simulink model "Gen_net_5"  (R2018b)
settings: Solver=FixedStepAuto  StartTime=0.0  StopTime=100  FixedStep=0.1  RelTol=1e-3
undefined symbols (not defined in the file): g, Jx, Jy, Jz, m, phi_DoS_duration_1, phi_DoS_duration_2, phi_DoS_duration_3, phi_DoS_duration_4, phi_DoS_duration_5, phi_FDI_value_1, phi_FDI_value_2, phi_FDI_value_3, phi_FDI_value_4, phi_FDI_value_5, phi_Replay_delay_1, phi_Replay_delay_2, phi_Replay_delay_3, phi_Replay_delay_4, phi_Replay_delay_5, psi_DoS_duration_1, psi_DoS_duration_2, psi_DoS_duration_3, psi_DoS_duration_4, psi_DoS_duration_5, psi_FDI_value_1, psi_FDI_value_2, psi_FDI_value_3, psi_FDI_value_4, psi_FDI_value_5, psi_Replay_delay_1, psi_Replay_delay_2, psi_Replay_delay_3, psi_Replay_delay_4, psi_Replay_delay_5, T_DoS_duration_1, T_DoS_duration_2, T_DoS_duration_3, T_DoS_duration_4, T_DoS_duration_5, T_FDI_value_1, T_FDI_value_2, T_FDI_value_3, T_FDI_value_4, T_FDI_value_5, T_Replay_delay_1, T_Replay_delay_2, T_Replay_delay_3, T_Replay_delay_4, T_Replay_delay_5, tau_phi_DoS_duration_1, tau_phi_DoS_duration_2, tau_phi_DoS_duration_3, tau_phi_DoS_duration_4, tau_phi_DoS_duration_5, tau_phi_FDI_value_1, tau_phi_FDI_value_2, tau_phi_FDI_value_3, tau_phi_FDI_value_4, tau_phi_FDI_value_5 ... (+95)
libraries: simulink x30
(part 1 of 4)
settings Model: Creator=afsha  LastModifiedBy=afsha
settings DataIOCC: ReturnWorkspaceOutputs=on  ReturnWorkspaceOutputsName=logsout

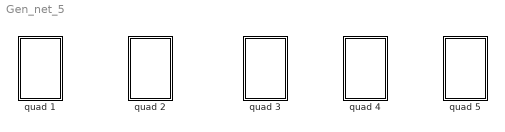
== system Gen_net_5 ==
  quad 1 : Subsystem
  quad 2 : Subsystem
  quad 3 : Subsystem
  quad 4 : Subsystem
  quad 5 : Subsystem

== system Gen_net_5/quad 1 ==
  actuator attack : Subsystem
  controller : Subsystem
  quadcopter : Subsystem
  references : Subsystem
  sensor attack : Subsystem
  wires:
  controller/4(tau_psi) -> actuator attack/4(tau_psi)  "tau_psi_1"
  quadcopter/4(phi) -> sensor attack/4(phi)  "phi"
  quadcopter/2(y) -> sensor attack/2(y)  "y"
  quadcopter/6(psi) -> sensor attack/6(psi)  "psi"
  references/2(y_ref) -> controller/2(y_ref)
  references/1(x_ref) -> controller/1(x_ref)
  controller/2(tau_phi) -> actuator attack/2(tau_phi)  "tau_phi_1"
  quadcopter/3(z) -> sensor attack/3(z)  "z"
  actuator attack/1(T_a) -> quadcopter/1(T)
  actuator attack/4(tau_psi_a) -> quadcopter/4(tau_psi)
  sensor attack/2(y_a) -> controller/5(y)  "y_a_1"
  sensor attack/4(phi_a) -> controller/7(phi)  "phi_a_1"
  quadcopter/1(x) -> sensor attack/1(x)  "x"
  actuator attack/3(tau_theta_a) -> quadcopter/3(tau_theta)
  sensor attack/5(theta_a) -> controller/8(theta)  "theta_a_1"
  sensor attack/6(psi_a) -> controller/9(psi)  "psi_a_1"
  controller/1(T) -> actuator attack/1(T)  "T_1"
  references/3(z_ref) -> controller/3(z_ref)
  controller/3(tau_theta) -> actuator attack/3(tau_theta)  "tau_theta_1"
  actuator attack/2(tau_phi_a) -> quadcopter/2(tau_ phi)
  sensor attack/1(x_a) -> controller/4(x)  "x_a_1"
  sensor attack/3(z_a) -> controller/6(z)  "z_a_1"
  quadcopter/5(theta) -> sensor attack/5(theta)  "theta"

== system Gen_net_5/quad 2 ==
  actuator attack : Subsystem
  controller : Subsystem
  quadcopter : Subsystem
  references : Subsystem
  sensor attack : Subsystem
  wires:
  controller/4(tau_psi) -> actuator attack/4(tau_psi)  "tau_psi_2"
  quadcopter/4(phi) -> sensor attack/4(phi)  "phi"
  quadcopter/2(y) -> sensor attack/2(y)  "y"
  quadcopter/6(psi) -> sensor attack/6(psi)  "psi"
  references/2(y_ref) -> controller/2(y_ref)
  references/1(x_ref) -> controller/1(x_ref)
  controller/2(tau_phi) -> actuator attack/2(tau_phi)  "tau_phi_2"
  quadcopter/3(z) -> sensor attack/3(z)  "z"
  actuator attack/1(T_a) -> quadcopter/1(T)
  actuator attack/4(tau_psi_a) -> quadcopter/4(tau_psi)
  sensor attack/2(y_a) -> controller/5(y)  "y_a_2"
  sensor attack/4(phi_a) -> controller/7(phi)  "phi_a_2"
  quadcopter/1(x) -> sensor attack/1(x)  "x"
  actuator attack/3(tau_theta_a) -> quadcopter/3(tau_theta)
  sensor attack/5(theta_a) -> controller/8(theta)  "theta_a_2"
  sensor attack/6(psi_a) -> controller/9(psi)  "psi_a_2"
  controller/1(T) -> actuator attack/1(T)  "T_2"
  references/3(z_ref) -> controller/3(z_ref)
  controller/3(tau_theta) -> actuator attack/3(tau_theta)  "tau_theta_2"
  actuator attack/2(tau_phi_a) -> quadcopter/2(tau_ phi)
  sensor attack/1(x_a) -> controller/4(x)  "x_a_2"
  sensor attack/3(z_a) -> controller/6(z)  "z_a_2"
  quadcopter/5(theta) -> sensor attack/5(theta)  "theta"

== system Gen_net_5/quad 3 ==
  actuator attack : Subsystem
  controller : Subsystem
  quadcopter : Subsystem
  references : Subsystem
  sensor attack : Subsystem
  wires:
  controller/4(tau_psi) -> actuator attack/4(tau_psi)  "tau_psi_3"
  quadcopter/4(phi) -> sensor attack/4(phi)  "phi"
  quadcopter/2(y) -> sensor attack/2(y)  "y"
  quadcopter/6(psi) -> sensor attack/6(psi)  "psi"
  references/2(y_ref) -> controller/2(y_ref)
  references/1(x_ref) -> controller/1(x_ref)
  controller/2(tau_phi) -> actuator attack/2(tau_phi)  "tau_phi_3"
  quadcopter/3(z) -> sensor attack/3(z)  "z"
  actuator attack/1(T_a) -> quadcopter/1(T)
  actuator attack/4(tau_psi_a) -> quadcopter/4(tau_psi)
  sensor attack/2(y_a) -> controller/5(y)  "y_a_3"
  sensor attack/4(phi_a) -> controller/7(phi)  "phi_a_3"
  quadcopter/1(x) -> sensor attack/1(x)  "x"
  actuator attack/3(tau_theta_a) -> quadcopter/3(tau_theta)
  sensor attack/5(theta_a) -> controller/8(theta)  "theta_a_3"
  sensor attack/6(psi_a) -> controller/9(psi)  "psi_a_3"
  controller/1(T) -> actuator attack/1(T)  "T_3"
  references/3(z_ref) -> controller/3(z_ref)
  controller/3(tau_theta) -> actuator attack/3(tau_theta)  "tau_theta_3"
  actuator attack/2(tau_phi_a) -> quadcopter/2(tau_ phi)
  sensor attack/1(x_a) -> controller/4(x)  "x_a_3"
  sensor attack/3(z_a) -> controller/6(z)  "z_a_3"
  quadcopter/5(theta) -> sensor attack/5(theta)  "theta"

== system Gen_net_5/quad 4 ==
  actuator attack : Subsystem
  controller : Subsystem
  quadcopter : Subsystem
  references : Subsystem
  sensor attack : Subsystem
  wires:
  controller/4(tau_psi) -> actuator attack/4(tau_psi)  "tau_psi_4"
  quadcopter/4(phi) -> sensor attack/4(phi)  "phi"
  quadcopter/2(y) -> sensor attack/2(y)  "y"
  quadcopter/6(psi) -> sensor attack/6(psi)  "psi"
  references/2(y_ref) -> controller/2(y_ref)
  references/1(x_ref) -> controller/1(x_ref)
  controller/2(tau_phi) -> actuator attack/2(tau_phi)  "tau_phi_4"
  quadcopter/3(z) -> sensor attack/3(z)  "z"
  actuator attack/1(T_a) -> quadcopter/1(T)
  actuator attack/4(tau_psi_a) -> quadcopter/4(tau_psi)
  sensor attack/2(y_a) -> controller/5(y)  "y_a_4"
  sensor attack/4(phi_a) -> controller/7(phi)  "phi_a_4"
  quadcopter/1(x) -> sensor attack/1(x)  "x"
  actuator attack/3(tau_theta_a) -> quadcopter/3(tau_theta)
  sensor attack/5(theta_a) -> controller/8(theta)  "theta_a_4"
  sensor attack/6(psi_a) -> controller/9(psi)  "psi_a_4"
  controller/1(T) -> actuator attack/1(T)  "T_4"
  references/3(z_ref) -> controller/3(z_ref)
  controller/3(tau_theta) -> actuator attack/3(tau_theta)  "tau_theta_4"
  actuator attack/2(tau_phi_a) -> quadcopter/2(tau_ phi)
  sensor attack/1(x_a) -> controller/4(x)  "x_a_4"
  sensor attack/3(z_a) -> controller/6(z)  "z_a_4"
  quadcopter/5(theta) -> sensor attack/5(theta)  "theta"

== system Gen_net_5/quad 5 ==
  actuator attack : Subsystem
  controller : Subsystem
  quadcopter : Subsystem
  references : Subsystem
  sensor attack : Subsystem
  wires:
  controller/4(tau_psi) -> actuator attack/4(tau_psi)  "tau_psi_5"
  quadcopter/4(phi) -> sensor attack/4(phi)  "phi"
  quadcopter/2(y) -> sensor attack/2(y)  "y"
  quadcopter/6(psi) -> sensor attack/6(psi)  "psi"
  references/2(y_ref) -> controller/2(y_ref)
  references/1(x_ref) -> controller/1(x_ref)
  controller/2(tau_phi) -> actuator attack/2(tau_phi)  "tau_phi_5"
  quadcopter/3(z) -> sensor attack/3(z)  "z"
  actuator attack/1(T_a) -> quadcopter/1(T)
  actuator attack/4(tau_psi_a) -> quadcopter/4(tau_psi)
  sensor attack/2(y_a) -> controller/5(y)  "y_a_5"
  sensor attack/4(phi_a) -> controller/7(phi)  "phi_a_5"
  quadcopter/1(x) -> sensor attack/1(x)  "x"
  actuator attack/3(tau_theta_a) -> quadcopter/3(tau_theta)
  sensor attack/5(theta_a) -> controller/8(theta)  "theta_a_5"
  sensor attack/6(psi_a) -> controller/9(psi)  "psi_a_5"
  controller/1(T) -> actuator attack/1(T)  "T_5"
  references/3(z_ref) -> controller/3(z_ref)
  controller/3(tau_theta) -> actuator attack/3(tau_theta)  "tau_theta_5"
  actuator attack/2(tau_phi_a) -> quadcopter/2(tau_ phi)
  sensor attack/1(x_a) -> controller/4(x)  "x_a_5"
  sensor attack/3(z_a) -> controller/6(z)  "z_a_5"
  quadcopter/5(theta) -> sensor attack/5(theta)  "theta"

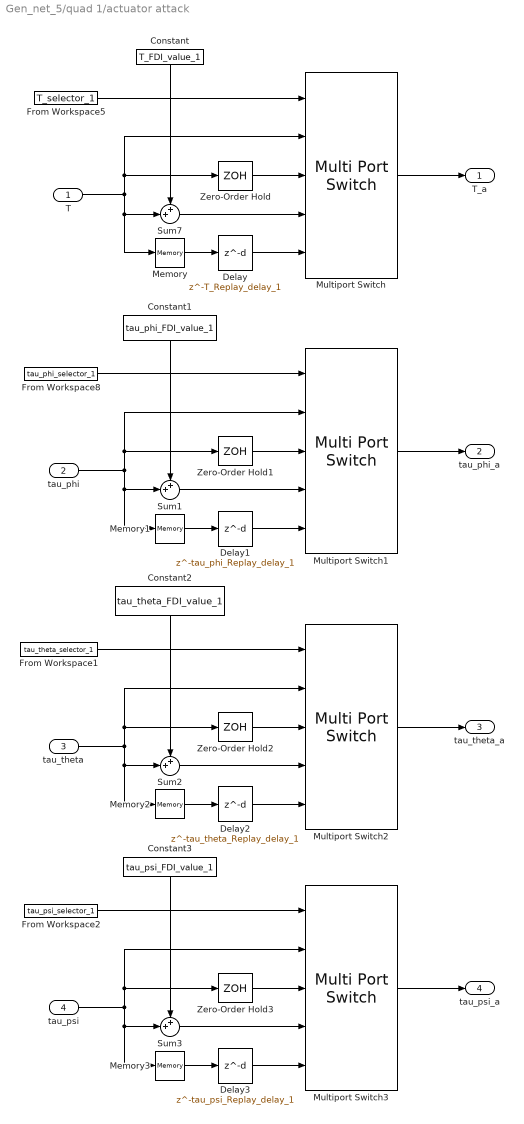
== system Gen_net_5/quad 1/actuator attack ==
  T : Inport
  tau_phi : Inport  Port=2
  tau_theta : Inport  Port=3
  tau_psi : Inport  Port=4
  Constant : Constant  Value=T_FDI_value_1
  Constant1 : Constant  Value=tau_phi_FDI_value_1
  Constant2 : Constant  Value=tau_theta_FDI_value_1
  Constant3 : Constant  Value=tau_psi_FDI_value_1
  Delay : Delay  DelayLength=T_Replay_delay_1  DelayLengthUpperLimit=40
  Delay1 : Delay  DelayLength=tau_phi_Replay_delay_1  DelayLengthUpperLimit=40
  Delay2 : Delay  DelayLength=tau_theta_Replay_delay_1  DelayLengthUpperLimit=40
  Delay3 : Delay  DelayLength=tau_psi_Replay_delay_1  DelayLengthUpperLimit=40
  From Workspace1 : FromWorkspace  VariableName=tau_theta_selector_1  SampleTime=0
  From Workspace2 : FromWorkspace  VariableName=tau_psi_selector_1  SampleTime=0
  From Workspace5 : FromWorkspace  VariableName=T_selector_1  SampleTime=0
  From Workspace8 : FromWorkspace  VariableName=tau_phi_selector_1  SampleTime=0
  Memory{,1..3} (4 alike) : Memory
  Multiport Switch{,1..3} (4 alike) : MultiPortSwitch  Inputs=4
  Sum{1..3,7} (4 alike) : Sum  Inputs=++|
  Zero-Order Hold : ZeroOrderHold  SampleTime=T_DoS_duration_1
  Zero-Order Hold1 : ZeroOrderHold  SampleTime=tau_phi_DoS_duration_1
  Zero-Order Hold2 : ZeroOrderHold  SampleTime=tau_theta_DoS_duration_1
  Zero-Order Hold3 : ZeroOrderHold  SampleTime=tau_psi_DoS_duration_1
  T_a : Outport
  tau_phi_a : Outport  Port=2
  tau_theta_a : Outport  Port=3
  tau_psi_a : Outport  Port=4
  wires:
  T/1 -> Sum7/2, Memory/1, Multiport Switch/2, Zero-Order Hold/1
  Zero-Order Hold/1 -> Multiport Switch/3
  Sum7/1 -> Multiport Switch/4
  From Workspace5/1 -> Multiport Switch/1
  Multiport Switch/1 -> T_a/1
  Memory/1 -> Delay/1
  Constant/1 -> Sum7/1
  Delay/1 -> Multiport Switch/5
  Memory1/1 -> Delay1/1
  Delay1/1 -> Multiport Switch1/5
  Zero-Order Hold1/1 -> Multiport Switch1/3
  Constant1/1 -> Sum1/1
  Sum1/1 -> Multiport Switch1/4
  Multiport Switch1/1 -> tau_phi_a/1
  tau_phi/1 -> Sum1/2, Memory1/1, Multiport Switch1/2, Zero-Order Hold1/1
  From Workspace8/1 -> Multiport Switch1/1
  Memory2/1 -> Delay2/1
  Delay2/1 -> Multiport Switch2/5
  Zero-Order Hold2/1 -> Multiport Switch2/3
  Constant2/1 -> Sum2/1
  Sum2/1 -> Multiport Switch2/4
  Multiport Switch2/1 -> tau_theta_a/1
  tau_theta/1 -> Sum2/2, Memory2/1, Multiport Switch2/2, Zero-Order Hold2/1
  From Workspace1/1 -> Multiport Switch2/1
  Memory3/1 -> Delay3/1
  Delay3/1 -> Multiport Switch3/5
  Zero-Order Hold3/1 -> Multiport Switch3/3
  Constant3/1 -> Sum3/1
  Sum3/1 -> Multiport Switch3/4
  Multiport Switch3/1 -> tau_psi_a/1
  tau_psi/1 -> Sum3/2, Memory3/1, Multiport Switch3/2, Zero-Order Hold3/1
  From Workspace2/1 -> Multiport Switch3/1

== system Gen_net_5/quad 1/controller ==
  x_ref : Inport
  y_ref : Inport  Port=2
  z_ref : Inport  Port=3
  x : Inport  Port=4
  y : Inport  Port=5
  z : Inport  Port=6
  phi : Inport  Port=7
  theta : Inport  Port=8
  psi : Inport  Port=9
  altitude controller : Subsystem
  attitude controller : Subsystem
  position controller : Subsystem
  yaw controller : Subsystem
  T : Outport
  tau_phi : Outport  Port=2
  tau_theta : Outport  Port=3
  tau_psi : Outport  Port=4
  wires:
  yaw controller/1(tau_psi) -> tau_psi/1
  phi/1 -> attitude controller/1(phi)
  y_ref/1 -> position controller/3(y_ref)
  x/1 -> position controller/2(x)
  position controller/2(theta_ref) -> attitude controller/4(theta_ref)
  position controller/1(phi_ref) -> attitude controller/3(phi_ref)
  x_ref/1 -> position controller/1(x_ref)
  attitude controller/1(tau_phi) -> tau_phi/1
  y/1 -> position controller/4(y)
  psi/1 -> yaw controller/1(yaw)
  attitude controller/2(tau_theta) -> tau_theta/1
  theta/1 -> attitude controller/2(theta)
  z_ref/1 -> altitude controller/1(z_ref)
  altitude controller/1(T) -> T/1
  z/1 -> altitude controller/2(z)

== system Gen_net_5/quad 1/quadcopter ==
  T : Inport
  tau_ phi : Inport  Port=2
  tau_theta : Inport  Port=3
  tau_psi : Inport  Port=4
  Demux : Demux  Outputs=12
  Demux1 : Demux  Outputs=12
  Gain : Gain  Gain=1/m
  Integrator12 : Integrator
  Mux : Mux  Inputs=12
  S(10-12) : Subsystem
  S(4-6) : Subsystem
  S(7-9) : Subsystem
  Scope1 : Scope  NumInputPorts=3
  Scope2 : Scope  NumInputPorts=3
  Terminator : Terminator
  Terminator1 : Terminator
  Terminator2 : Terminator
  angle : Scope  NumInputPorts=3
  position : Scope  NumInputPorts=3
  x : Outport
  y : Outport  Port=2
  z : Outport  Port=3
  phi : Outport  Port=4
  theta : Outport  Port=5
  psi : Outport  Port=6
  wires:
  Mux/1 -> Integrator12/1
  Integrator12/1 -> Demux/1, Demux1/1
  Demux/2 -> position/2, y/1  "y"
  Demux/3 -> z/1, position/3  "z"
  Demux/1 -> x/1, position/1  "x"
  Demux/5 -> Scope1/2  "Vy"
  Demux/4 -> Scope1/1  "Vx"
  Demux/6 -> Scope1/3  "Vz"
  Demux/8 -> angle/2, theta/1  "theta"
  Demux/7 -> angle/1, phi/1  "phi"
  Demux/9 -> angle/3, psi/1  "psi"
  Demux/12 -> Scope2/3  "r"
  Demux/10 -> Scope2/1  "p"
  Demux/11 -> Scope2/2  "q"
  Demux1/4 -> Mux/1  "Vx"
  Demux1/5 -> Mux/2  "Vy"
  Demux1/6 -> Mux/3  "Vz"
  Demux1/8 -> S(4-6)/3(theta), S(7-9)/2(theta)  "theta"
  Demux1/7 -> S(4-6)/2(phi), S(7-9)/1(phi)  "phi"
  Demux1/10 -> S(10-12)/2(P), S(7-9)/4(P)  "P"
  Demux1/11 -> S(7-9)/3(q), S(10-12)/1(q)  "q"
  Demux1/12 -> S(7-9)/5(r), S(10-12)/3(r)
  Gain/1 -> S(4-6)/1(In1)
  Demux1/9 -> S(4-6)/4(psi)  "psi"
  S(4-6)/1(Out1) -> Mux/4
  S(4-6)/2(Out2) -> Mux/5
  S(4-6)/3(Out3) -> Mux/6
  S(7-9)/1(Out1) -> Mux/7
  S(7-9)/2(Out2) -> Mux/8
  S(7-9)/3(Out3) -> Mux/9
  tau_ phi/1 -> S(10-12)/4(In4)
  tau_theta/1 -> S(10-12)/5(In5)
  tau_psi/1 -> S(10-12)/6(In6)
  S(10-12)/1(Out1) -> Mux/10
  S(10-12)/2(Out2) -> Mux/11
  S(10-12)/3(Out3) -> Mux/12
  Demux1/1 -> Terminator/1  "x"
  Demux1/2 -> Terminator1/1  "y"
  Demux1/3 -> Terminator2/1  "z"
  T/1 -> Gain/1  "z_ref"

== system Gen_net_5/quad 1/references ==
  From Workspace : FromWorkspace  VariableName=z_ref_1  SampleTime=0
  From Workspace1 : FromWorkspace  VariableName=x_ref_1  SampleTime=0
  From Workspace2 : FromWorkspace  VariableName=y_ref_1  SampleTime=0
  reference : Scope  NumInputPorts=3
  x_ref : Outport
  y_ref : Outport  Port=2
  z_ref : Outport  Port=3
  wires:
  From Workspace1/1 -> reference/1, x_ref/1  "x_ref"
  From Workspace/1 -> reference/3, z_ref/1  "z_ref"
  From Workspace2/1 -> reference/2, y_ref/1  "y_ref"

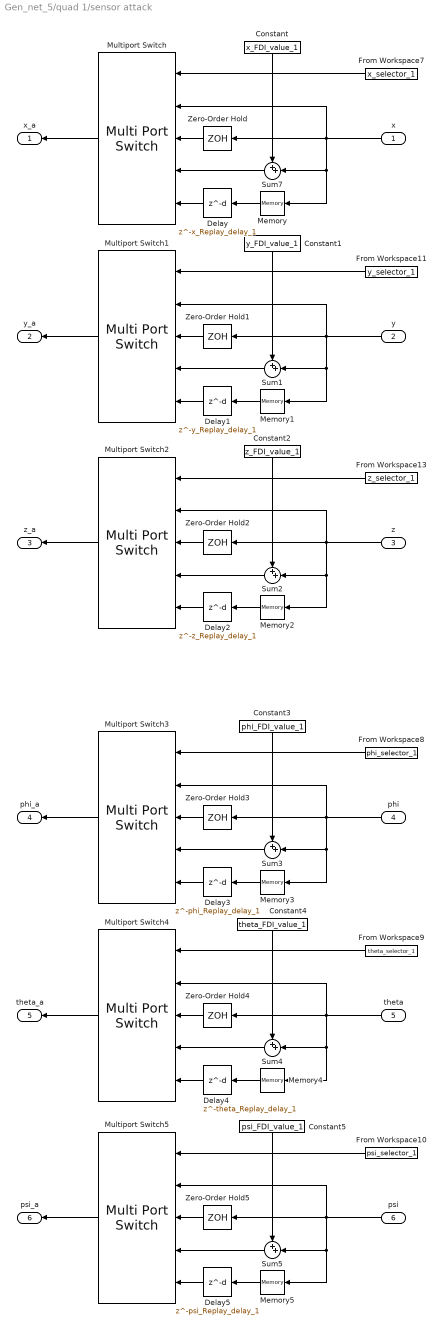
== system Gen_net_5/quad 1/sensor attack ==
  x : Inport
  y : Inport  Port=2
  z : Inport  Port=3
  phi : Inport  Port=4
  theta : Inport  Port=5
  psi : Inport  Port=6
  Constant : Constant  Value=x_FDI_value_1
  Constant1 : Constant  Value=y_FDI_value_1
  Constant2 : Constant  Value=z_FDI_value_1
  Constant3 : Constant  Value=phi_FDI_value_1
  Constant4 : Constant  Value=theta_FDI_value_1
  Constant5 : Constant  Value=psi_FDI_value_1
  Delay : Delay  DelayLength=x_Replay_delay_1  DelayLengthUpperLimit=40
  Delay1 : Delay  DelayLength=y_Replay_delay_1  DelayLengthUpperLimit=40
  Delay2 : Delay  DelayLength=z_Replay_delay_1  DelayLengthUpperLimit=40
  Delay3 : Delay  DelayLength=phi_Replay_delay_1  DelayLengthUpperLimit=40
  Delay4 : Delay  DelayLength=theta_Replay_delay_1  DelayLengthUpperLimit=40
  Delay5 : Delay  DelayLength=psi_Replay_delay_1  DelayLengthUpperLimit=40
  From Workspace10 : FromWorkspace  VariableName=psi_selector_1  SampleTime=0
  From Workspace11 : FromWorkspace  VariableName=y_selector_1  SampleTime=0
  From Workspace13 : FromWorkspace  VariableName=z_selector_1  SampleTime=0
  From Workspace7 : FromWorkspace  VariableName=x_selector_1  SampleTime=0
  From Workspace8 : FromWorkspace  VariableName=phi_selector_1  SampleTime=0
  From Workspace9 : FromWorkspace  VariableName=theta_selector_1  SampleTime=0
  Memory{,1..5} (6 alike) : Memory
  Multiport Switch{,1..5} (6 alike) : MultiPortSwitch  Inputs=4
  Sum{1..5,7} (6 alike) : Sum  Inputs=++|
  Zero-Order Hold : ZeroOrderHold  SampleTime=x_DoS_duration_1
  Zero-Order Hold1 : ZeroOrderHold  SampleTime=y_DoS_duration_1
  Zero-Order Hold2 : ZeroOrderHold  SampleTime=z_DoS_duration_1
  Zero-Order Hold3 : ZeroOrderHold  SampleTime=phi_DoS_duration_1
  Zero-Order Hold4 : ZeroOrderHold  SampleTime=theta_DoS_duration_1
  Zero-Order Hold5 : ZeroOrderHold  SampleTime=psi_DoS_duration_1
  x_a : Outport
  y_a : Outport  Port=2
  z_a : Outport  Port=3
  phi_a : Outport  Port=4
  theta_a : Outport  Port=5
  psi_a : Outport  Port=6
  wires:
  Memory/1 -> Delay/1
  Delay/1 -> Multiport Switch/5
  Zero-Order Hold/1 -> Multiport Switch/3
  Constant/1 -> Sum7/1
  Sum7/1 -> Multiport Switch/4
  Multiport Switch/1 -> x_a/1
  x/1 -> Multiport Switch/2, Zero-Order Hold/1, Sum7/2, Memory/1
  From Workspace7/1 -> Multiport Switch/1
  From Workspace11/1 -> Multiport Switch1/1
  Sum1/1 -> Multiport Switch1/4
  Delay1/1 -> Multiport Switch1/5
  Constant1/1 -> Sum1/1
  Memory1/1 -> Delay1/1
  y/1 -> Multiport Switch1/2, Zero-Order Hold1/1, Sum1/2, Memory1/1
  Multiport Switch1/1 -> y_a/1
  Zero-Order Hold1/1 -> Multiport Switch1/3
  From Workspace13/1 -> Multiport Switch2/1
  Sum2/1 -> Multiport Switch2/4
  Delay2/1 -> Multiport Switch2/5
  Constant2/1 -> Sum2/1
  Memory2/1 -> Delay2/1
  z/1 -> Multiport Switch2/2, Zero-Order Hold2/1, Sum2/2, Memory2/1
  Multiport Switch2/1 -> z_a/1
  Zero-Order Hold2/1 -> Multiport Switch2/3
  From Workspace8/1 -> Multiport Switch3/1
  Sum3/1 -> Multiport Switch3/4
  Delay3/1 -> Multiport Switch3/5
  Constant3/1 -> Sum3/1
  Memory3/1 -> Delay3/1
  phi/1 -> Multiport Switch3/2, Zero-Order Hold3/1, Sum3/2, Memory3/1
  Multiport Switch3/1 -> phi_a/1
  Zero-Order Hold3/1 -> Multiport Switch3/3
  From Workspace9/1 -> Multiport Switch4/1
  Sum4/1 -> Multiport Switch4/4
  Delay4/1 -> Multiport Switch4/5
  Constant4/1 -> Sum4/1
  Memory4/1 -> Delay4/1
  theta/1 -> Multiport Switch4/2, Zero-Order Hold4/1, Sum4/2, Memory4/1
  Multiport Switch4/1 -> theta_a/1
  Zero-Order Hold4/1 -> Multiport Switch4/3
  From Workspace10/1 -> Multiport Switch5/1
  Sum5/1 -> Multiport Switch5/4
  Delay5/1 -> Multiport Switch5/5
  Constant5/1 -> Sum5/1
  Memory5/1 -> Delay5/1
  psi/1 -> Multiport Switch5/2, Zero-Order Hold5/1, Sum5/2, Memory5/1
  Multiport Switch5/1 -> psi_a/1
  Zero-Order Hold5/1 -> Multiport Switch5/3

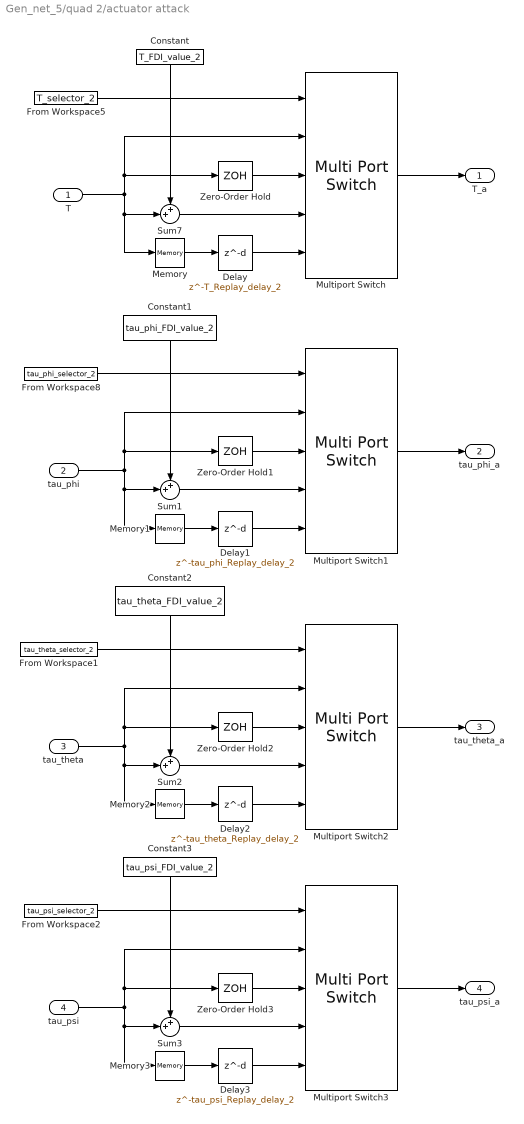
== system Gen_net_5/quad 2/actuator attack ==
  T : Inport
  tau_phi : Inport  Port=2
  tau_theta : Inport  Port=3
  tau_psi : Inport  Port=4
  Constant : Constant  Value=T_FDI_value_2
  Constant1 : Constant  Value=tau_phi_FDI_value_2
  Constant2 : Constant  Value=tau_theta_FDI_value_2
  Constant3 : Constant  Value=tau_psi_FDI_value_2
  Delay : Delay  DelayLength=T_Replay_delay_2  DelayLengthUpperLimit=40
  Delay1 : Delay  DelayLength=tau_phi_Replay_delay_2  DelayLengthUpperLimit=40
  Delay2 : Delay  DelayLength=tau_theta_Replay_delay_2  DelayLengthUpperLimit=40
  Delay3 : Delay  DelayLength=tau_psi_Replay_delay_2  DelayLengthUpperLimit=40
  From Workspace1 : FromWorkspace  VariableName=tau_theta_selector_2  SampleTime=0
  From Workspace2 : FromWorkspace  VariableName=tau_psi_selector_2  SampleTime=0
  From Workspace5 : FromWorkspace  VariableName=T_selector_2  SampleTime=0
  From Workspace8 : FromWorkspace  VariableName=tau_phi_selector_2  SampleTime=0
  Memory{,1..3} (4 alike) : Memory
  Multiport Switch{,1..3} (4 alike) : MultiPortSwitch  Inputs=4
  Sum{1..3,7} (4 alike) : Sum  Inputs=++|
  Zero-Order Hold : ZeroOrderHold  SampleTime=T_DoS_duration_2
  Zero-Order Hold1 : ZeroOrderHold  SampleTime=tau_phi_DoS_duration_2
  Zero-Order Hold2 : ZeroOrderHold  SampleTime=tau_theta_DoS_duration_2
  Zero-Order Hold3 : ZeroOrderHold  SampleTime=tau_psi_DoS_duration_2
  T_a : Outport
  tau_phi_a : Outport  Port=2
  tau_theta_a : Outport  Port=3
  tau_psi_a : Outport  Port=4
  wires:
  T/1 -> Sum7/2, Memory/1, Multiport Switch/2, Zero-Order Hold/1
  Zero-Order Hold/1 -> Multiport Switch/3
  Sum7/1 -> Multiport Switch/4
  From Workspace5/1 -> Multiport Switch/1
  Multiport Switch/1 -> T_a/1
  Memory/1 -> Delay/1
  Constant/1 -> Sum7/1
  Delay/1 -> Multiport Switch/5
  Memory1/1 -> Delay1/1
  Delay1/1 -> Multiport Switch1/5
  Zero-Order Hold1/1 -> Multiport Switch1/3
  Constant1/1 -> Sum1/1
  Sum1/1 -> Multiport Switch1/4
  Multiport Switch1/1 -> tau_phi_a/1
  tau_phi/1 -> Sum1/2, Memory1/1, Multiport Switch1/2, Zero-Order Hold1/1
  From Workspace8/1 -> Multiport Switch1/1
  Memory2/1 -> Delay2/1
  Delay2/1 -> Multiport Switch2/5
  Zero-Order Hold2/1 -> Multiport Switch2/3
  Constant2/1 -> Sum2/1
  Sum2/1 -> Multiport Switch2/4
  Multiport Switch2/1 -> tau_theta_a/1
  tau_theta/1 -> Sum2/2, Memory2/1, Multiport Switch2/2, Zero-Order Hold2/1
  From Workspace1/1 -> Multiport Switch2/1
  Memory3/1 -> Delay3/1
  Delay3/1 -> Multiport Switch3/5
  Zero-Order Hold3/1 -> Multiport Switch3/3
  Constant3/1 -> Sum3/1
  Sum3/1 -> Multiport Switch3/4
  Multiport Switch3/1 -> tau_psi_a/1
  tau_psi/1 -> Sum3/2, Memory3/1, Multiport Switch3/2, Zero-Order Hold3/1
  From Workspace2/1 -> Multiport Switch3/1

== system Gen_net_5/quad 2/controller ==
  x_ref : Inport
  y_ref : Inport  Port=2
  z_ref : Inport  Port=3
  x : Inport  Port=4
  y : Inport  Port=5
  z : Inport  Port=6
  phi : Inport  Port=7
  theta : Inport  Port=8
  psi : Inport  Port=9
  altitude controller : Subsystem
  attitude controller : Subsystem
  position controller : Subsystem
  yaw controller : Subsystem
  T : Outport
  tau_phi : Outport  Port=2
  tau_theta : Outport  Port=3
  tau_psi : Outport  Port=4
  wires:
  yaw controller/1(tau_psi) -> tau_psi/1
  phi/1 -> attitude controller/1(phi)
  y_ref/1 -> position controller/3(y_ref)
  x/1 -> position controller/2(x)
  position controller/2(theta_ref) -> attitude controller/4(theta_ref)
  position controller/1(phi_ref) -> attitude controller/3(phi_ref)
  x_ref/1 -> position controller/1(x_ref)
  attitude controller/1(tau_phi) -> tau_phi/1
  y/1 -> position controller/4(y)
  psi/1 -> yaw controller/1(yaw)
  attitude controller/2(tau_theta) -> tau_theta/1
  theta/1 -> attitude controller/2(theta)
  z_ref/1 -> altitude controller/1(z_ref)
  altitude controller/1(T) -> T/1
  z/1 -> altitude controller/2(z)

== system Gen_net_5/quad 2/quadcopter ==
  T : Inport
  tau_ phi : Inport  Port=2
  tau_theta : Inport  Port=3
  tau_psi : Inport  Port=4
  Demux : Demux  Outputs=12
  Demux1 : Demux  Outputs=12
  Gain : Gain  Gain=1/m
  Integrator12 : Integrator
  Mux : Mux  Inputs=12
  S(10-12) : Subsystem
  S(4-6) : Subsystem
  S(7-9) : Subsystem
  Scope1 : Scope  NumInputPorts=3
  Scope2 : Scope  NumInputPorts=3
  Terminator : Terminator
  Terminator1 : Terminator
  Terminator2 : Terminator
  angle : Scope  NumInputPorts=3
  position : Scope  NumInputPorts=3
  x : Outport
  y : Outport  Port=2
  z : Outport  Port=3
  phi : Outport  Port=4
  theta : Outport  Port=5
  psi : Outport  Port=6
  wires:
  Mux/1 -> Integrator12/1
  Integrator12/1 -> Demux/1, Demux1/1
  Demux/2 -> position/2, y/1  "y"
  Demux/3 -> z/1, position/3  "z"
  Demux/1 -> x/1, position/1  "x"
  Demux/5 -> Scope1/2  "Vy"
  Demux/4 -> Scope1/1  "Vx"
  Demux/6 -> Scope1/3  "Vz"
  Demux/8 -> angle/2, theta/1  "theta"
  Demux/7 -> angle/1, phi/1  "phi"
  Demux/9 -> angle/3, psi/1  "psi"
  Demux/12 -> Scope2/3  "r"
  Demux/10 -> Scope2/1  "p"
  Demux/11 -> Scope2/2  "q"
  Demux1/4 -> Mux/1  "Vx"
  Demux1/5 -> Mux/2  "Vy"
  Demux1/6 -> Mux/3  "Vz"
  Demux1/8 -> S(4-6)/3(theta), S(7-9)/2(theta)  "theta"
  Demux1/7 -> S(4-6)/2(phi), S(7-9)/1(phi)  "phi"
  Demux1/10 -> S(10-12)/2(P), S(7-9)/4(P)  "P"
  Demux1/11 -> S(7-9)/3(q), S(10-12)/1(q)  "q"
  Demux1/12 -> S(7-9)/5(r), S(10-12)/3(r)
  Gain/1 -> S(4-6)/1(In1)
  Demux1/9 -> S(4-6)/4(psi)  "psi"
  S(4-6)/1(Out1) -> Mux/4
  S(4-6)/2(Out2) -> Mux/5
  S(4-6)/3(Out3) -> Mux/6
  S(7-9)/1(Out1) -> Mux/7
  S(7-9)/2(Out2) -> Mux/8
  S(7-9)/3(Out3) -> Mux/9
  tau_ phi/1 -> S(10-12)/4(In4)
  tau_theta/1 -> S(10-12)/5(In5)
  tau_psi/1 -> S(10-12)/6(In6)
  S(10-12)/1(Out1) -> Mux/10
  S(10-12)/2(Out2) -> Mux/11
  S(10-12)/3(Out3) -> Mux/12
  Demux1/1 -> Terminator/1  "x"
  Demux1/2 -> Terminator1/1  "y"
  Demux1/3 -> Terminator2/1  "z"
  T/1 -> Gain/1  "z_ref"

== system Gen_net_5/quad 2/references ==
  From Workspace : FromWorkspace  VariableName=z_ref_2  SampleTime=0
  From Workspace1 : FromWorkspace  VariableName=x_ref_2  SampleTime=0
  From Workspace2 : FromWorkspace  VariableName=y_ref_2  SampleTime=0
  reference : Scope  NumInputPorts=3
  x_ref : Outport
  y_ref : Outport  Port=2
  z_ref : Outport  Port=3
  wires:
  From Workspace1/1 -> reference/1, x_ref/1  "x_ref"
  From Workspace/1 -> reference/3, z_ref/1  "z_ref"
  From Workspace2/1 -> reference/2, y_ref/1  "y_ref"

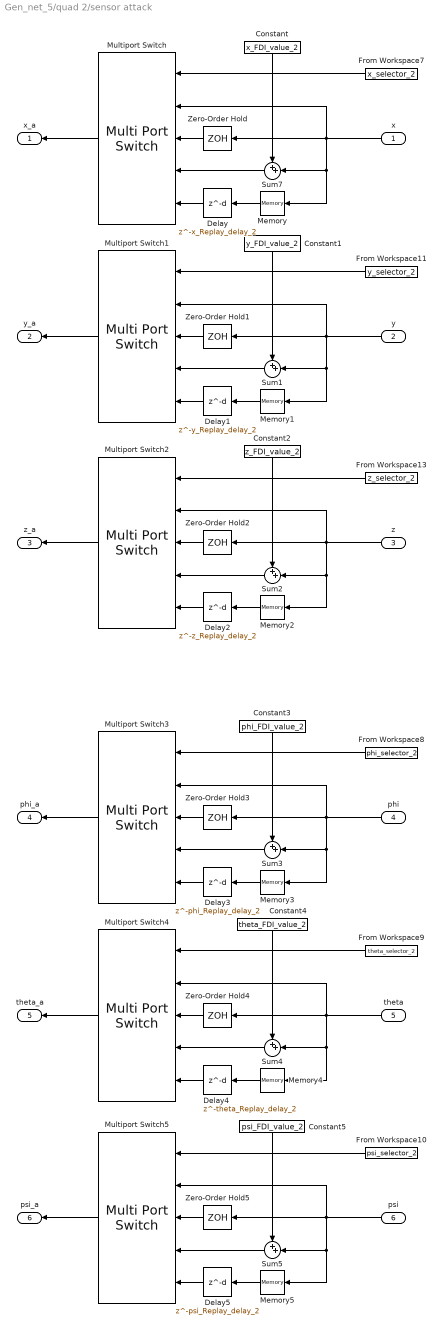
== system Gen_net_5/quad 2/sensor attack ==
  x : Inport
  y : Inport  Port=2
  z : Inport  Port=3
  phi : Inport  Port=4
  theta : Inport  Port=5
  psi : Inport  Port=6
  Constant : Constant  Value=x_FDI_value_2
  Constant1 : Constant  Value=y_FDI_value_2
  Constant2 : Constant  Value=z_FDI_value_2
  Constant3 : Constant  Value=phi_FDI_value_2
  Constant4 : Constant  Value=theta_FDI_value_2
  Constant5 : Constant  Value=psi_FDI_value_2
  Delay : Delay  DelayLength=x_Replay_delay_2  DelayLengthUpperLimit=40
  Delay1 : Delay  DelayLength=y_Replay_delay_2  DelayLengthUpperLimit=40
  Delay2 : Delay  DelayLength=z_Replay_delay_2  DelayLengthUpperLimit=40
  Delay3 : Delay  DelayLength=phi_Replay_delay_2  DelayLengthUpperLimit=40
  Delay4 : Delay  DelayLength=theta_Replay_delay_2  DelayLengthUpperLimit=40
  Delay5 : Delay  DelayLength=psi_Replay_delay_2  DelayLengthUpperLimit=40
  From Workspace10 : FromWorkspace  VariableName=psi_selector_2  SampleTime=0
  From Workspace11 : FromWorkspace  VariableName=y_selector_2  SampleTime=0
  From Workspace13 : FromWorkspace  VariableName=z_selector_2  SampleTime=0
  From Workspace7 : FromWorkspace  VariableName=x_selector_2  SampleTime=0
  From Workspace8 : FromWorkspace  VariableName=phi_selector_2  SampleTime=0
  From Workspace9 : FromWorkspace  VariableName=theta_selector_2  SampleTime=0
  Memory{,1..5} (6 alike) : Memory
  Multiport Switch{,1..5} (6 alike) : MultiPortSwitch  Inputs=4
  Sum{1..5,7} (6 alike) : Sum  Inputs=++|
  Zero-Order Hold : ZeroOrderHold  SampleTime=x_DoS_duration_2
  Zero-Order Hold1 : ZeroOrderHold  SampleTime=y_DoS_duration_2
  Zero-Order Hold2 : ZeroOrderHold  SampleTime=z_DoS_duration_2
  Zero-Order Hold3 : ZeroOrderHold  SampleTime=phi_DoS_duration_2
  Zero-Order Hold4 : ZeroOrderHold  SampleTime=theta_DoS_duration_2
  Zero-Order Hold5 : ZeroOrderHold  SampleTime=psi_DoS_duration_2
  x_a : Outport
  y_a : Outport  Port=2
  z_a : Outport  Port=3
  phi_a : Outport  Port=4
  theta_a : Outport  Port=5
  psi_a : Outport  Port=6
  wires:
  Memory/1 -> Delay/1
  Delay/1 -> Multiport Switch/5
  Zero-Order Hold/1 -> Multiport Switch/3
  Constant/1 -> Sum7/1
  Sum7/1 -> Multiport Switch/4
  Multiport Switch/1 -> x_a/1
  x/1 -> Multiport Switch/2, Zero-Order Hold/1, Sum7/2, Memory/1
  From Workspace7/1 -> Multiport Switch/1
  From Workspace11/1 -> Multiport Switch1/1
  Sum1/1 -> Multiport Switch1/4
  Delay1/1 -> Multiport Switch1/5
  Constant1/1 -> Sum1/1
  Memory1/1 -> Delay1/1
  y/1 -> Multiport Switch1/2, Zero-Order Hold1/1, Sum1/2, Memory1/1
  Multiport Switch1/1 -> y_a/1
  Zero-Order Hold1/1 -> Multiport Switch1/3
  From Workspace13/1 -> Multiport Switch2/1
  Sum2/1 -> Multiport Switch2/4
  Delay2/1 -> Multiport Switch2/5
  Constant2/1 -> Sum2/1
  Memory2/1 -> Delay2/1
  z/1 -> Multiport Switch2/2, Zero-Order Hold2/1, Sum2/2, Memory2/1
  Multiport Switch2/1 -> z_a/1
  Zero-Order Hold2/1 -> Multiport Switch2/3
  From Workspace8/1 -> Multiport Switch3/1
  Sum3/1 -> Multiport Switch3/4
  Delay3/1 -> Multiport Switch3/5
  Constant3/1 -> Sum3/1
  Memory3/1 -> Delay3/1
  phi/1 -> Multiport Switch3/2, Zero-Order Hold3/1, Sum3/2, Memory3/1
  Multiport Switch3/1 -> phi_a/1
  Zero-Order Hold3/1 -> Multiport Switch3/3
  From Workspace9/1 -> Multiport Switch4/1
  Sum4/1 -> Multiport Switch4/4
  Delay4/1 -> Multiport Switch4/5
  Constant4/1 -> Sum4/1
  Memory4/1 -> Delay4/1
  theta/1 -> Multiport Switch4/2, Zero-Order Hold4/1, Sum4/2, Memory4/1
  Multiport Switch4/1 -> theta_a/1
  Zero-Order Hold4/1 -> Multiport Switch4/3
  From Workspace10/1 -> Multiport Switch5/1
  Sum5/1 -> Multiport Switch5/4
  Delay5/1 -> Multiport Switch5/5
  Constant5/1 -> Sum5/1
  Memory5/1 -> Delay5/1
  psi/1 -> Multiport Switch5/2, Zero-Order Hold5/1, Sum5/2, Memory5/1
  Multiport Switch5/1 -> psi_a/1
  Zero-Order Hold5/1 -> Multiport Switch5/3

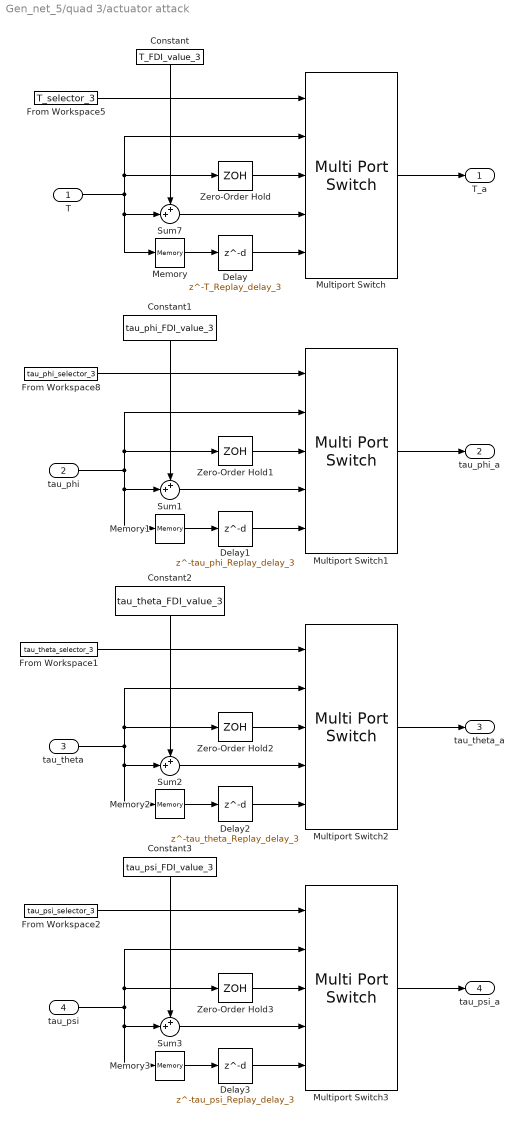
== system Gen_net_5/quad 3/actuator attack ==
  T : Inport
  tau_phi : Inport  Port=2
  tau_theta : Inport  Port=3
  tau_psi : Inport  Port=4
  Constant : Constant  Value=T_FDI_value_3
  Constant1 : Constant  Value=tau_phi_FDI_value_3
  Constant2 : Constant  Value=tau_theta_FDI_value_3
  Constant3 : Constant  Value=tau_psi_FDI_value_3
  Delay : Delay  DelayLength=T_Replay_delay_3  DelayLengthUpperLimit=40
  Delay1 : Delay  DelayLength=tau_phi_Replay_delay_3  DelayLengthUpperLimit=40
  Delay2 : Delay  DelayLength=tau_theta_Replay_delay_3  DelayLengthUpperLimit=40
  Delay3 : Delay  DelayLength=tau_psi_Replay_delay_3  DelayLengthUpperLimit=40
  From Workspace1 : FromWorkspace  VariableName=tau_theta_selector_3  SampleTime=0
  From Workspace2 : FromWorkspace  VariableName=tau_psi_selector_3  SampleTime=0
  From Workspace5 : FromWorkspace  VariableName=T_selector_3  SampleTime=0
  From Workspace8 : FromWorkspace  VariableName=tau_phi_selector_3  SampleTime=0
  Memory{,1..3} (4 alike) : Memory
  Multiport Switch{,1..3} (4 alike) : MultiPortSwitch  Inputs=4
  Sum{1..3,7} (4 alike) : Sum  Inputs=++|
  Zero-Order Hold : ZeroOrderHold  SampleTime=T_DoS_duration_3
  Zero-Order Hold1 : ZeroOrderHold  SampleTime=tau_phi_DoS_duration_3
  Zero-Order Hold2 : ZeroOrderHold  SampleTime=tau_theta_DoS_duration_3
  Zero-Order Hold3 : ZeroOrderHold  SampleTime=tau_psi_DoS_duration_3
  T_a : Outport
  tau_phi_a : Outport  Port=2
  tau_theta_a : Outport  Port=3
  tau_psi_a : Outport  Port=4
  wires:
  T/1 -> Sum7/2, Memory/1, Multiport Switch/2, Zero-Order Hold/1
  Zero-Order Hold/1 -> Multiport Switch/3
  Sum7/1 -> Multiport Switch/4
  From Workspace5/1 -> Multiport Switch/1
  Multiport Switch/1 -> T_a/1
  Memory/1 -> Delay/1
  Constant/1 -> Sum7/1
  Delay/1 -> Multiport Switch/5
  Memory1/1 -> Delay1/1
  Delay1/1 -> Multiport Switch1/5
  Zero-Order Hold1/1 -> Multiport Switch1/3
  Constant1/1 -> Sum1/1
  Sum1/1 -> Multiport Switch1/4
  Multiport Switch1/1 -> tau_phi_a/1
  tau_phi/1 -> Sum1/2, Memory1/1, Multiport Switch1/2, Zero-Order Hold1/1
  From Workspace8/1 -> Multiport Switch1/1
  Memory2/1 -> Delay2/1
  Delay2/1 -> Multiport Switch2/5
  Zero-Order Hold2/1 -> Multiport Switch2/3
  Constant2/1 -> Sum2/1
  Sum2/1 -> Multiport Switch2/4
  Multiport Switch2/1 -> tau_theta_a/1
  tau_theta/1 -> Sum2/2, Memory2/1, Multiport Switch2/2, Zero-Order Hold2/1
  From Workspace1/1 -> Multiport Switch2/1
  Memory3/1 -> Delay3/1
  Delay3/1 -> Multiport Switch3/5
  Zero-Order Hold3/1 -> Multiport Switch3/3
  Constant3/1 -> Sum3/1
  Sum3/1 -> Multiport Switch3/4
  Multiport Switch3/1 -> tau_psi_a/1
  tau_psi/1 -> Sum3/2, Memory3/1, Multiport Switch3/2, Zero-Order Hold3/1
  From Workspace2/1 -> Multiport Switch3/1

== system Gen_net_5/quad 3/controller ==
  x_ref : Inport
  y_ref : Inport  Port=2
  z_ref : Inport  Port=3
  x : Inport  Port=4
  y : Inport  Port=5
  z : Inport  Port=6
  phi : Inport  Port=7
  theta : Inport  Port=8
  psi : Inport  Port=9
  altitude controller : Subsystem
  attitude controller : Subsystem
  position controller : Subsystem
  yaw controller : Subsystem
  T : Outport
  tau_phi : Outport  Port=2
  tau_theta : Outport  Port=3
  tau_psi : Outport  Port=4
  wires:
  yaw controller/1(tau_psi) -> tau_psi/1
  phi/1 -> attitude controller/1(phi)
  y_ref/1 -> position controller/3(y_ref)
  x/1 -> position controller/2(x)
  position controller/2(theta_ref) -> attitude controller/4(theta_ref)
  position controller/1(phi_ref) -> attitude controller/3(phi_ref)
  x_ref/1 -> position controller/1(x_ref)
  attitude controller/1(tau_phi) -> tau_phi/1
  y/1 -> position controller/4(y)
  psi/1 -> yaw controller/1(yaw)
  attitude controller/2(tau_theta) -> tau_theta/1
  theta/1 -> attitude controller/2(theta)
  z_ref/1 -> altitude controller/1(z_ref)
  altitude controller/1(T) -> T/1
  z/1 -> altitude controller/2(z)

== system Gen_net_5/quad 3/quadcopter ==
  T : Inport
  tau_ phi : Inport  Port=2
  tau_theta : Inport  Port=3
  tau_psi : Inport  Port=4
  Demux : Demux  Outputs=12
  Demux1 : Demux  Outputs=12
  Gain : Gain  Gain=1/m
  Integrator12 : Integrator
  Mux : Mux  Inputs=12
  S(10-12) : Subsystem
  S(4-6) : Subsystem
  S(7-9) : Subsystem
  Scope1 : Scope  NumInputPorts=3
  Scope2 : Scope  NumInputPorts=3
  Terminator : Terminator
  Terminator1 : Terminator
  Terminator2 : Terminator
  angle : Scope  NumInputPorts=3
  position : Scope  NumInputPorts=3
  x : Outport
  y : Outport  Port=2
  z : Outport  Port=3
  phi : Outport  Port=4
  theta : Outport  Port=5
  psi : Outport  Port=6
  wires:
  Mux/1 -> Integrator12/1
  Integrator12/1 -> Demux/1, Demux1/1
  Demux/2 -> position/2, y/1  "y"
  Demux/3 -> z/1, position/3  "z"
  Demux/1 -> x/1, position/1  "x"
  Demux/5 -> Scope1/2  "Vy"
  Demux/4 -> Scope1/1  "Vx"
  Demux/6 -> Scope1/3  "Vz"
  Demux/8 -> angle/2, theta/1  "theta"
  Demux/7 -> angle/1, phi/1  "phi"
  Demux/9 -> angle/3, psi/1  "psi"
  Demux/12 -> Scope2/3  "r"
  Demux/10 -> Scope2/1  "p"
  Demux/11 -> Scope2/2  "q"
  Demux1/4 -> Mux/1  "Vx"
  Demux1/5 -> Mux/2  "Vy"
  Demux1/6 -> Mux/3  "Vz"
  Demux1/8 -> S(4-6)/3(theta), S(7-9)/2(theta)  "theta"
  Demux1/7 -> S(4-6)/2(phi), S(7-9)/1(phi)  "phi"
  Demux1/10 -> S(10-12)/2(P), S(7-9)/4(P)  "P"
  Demux1/11 -> S(7-9)/3(q), S(10-12)/1(q)  "q"
  Demux1/12 -> S(7-9)/5(r), S(10-12)/3(r)
  Gain/1 -> S(4-6)/1(In1)
  Demux1/9 -> S(4-6)/4(psi)  "psi"
  S(4-6)/1(Out1) -> Mux/4
  S(4-6)/2(Out2) -> Mux/5
  S(4-6)/3(Out3) -> Mux/6
  S(7-9)/1(Out1) -> Mux/7
  S(7-9)/2(Out2) -> Mux/8
  S(7-9)/3(Out3) -> Mux/9
  tau_ phi/1 -> S(10-12)/4(In4)
  tau_theta/1 -> S(10-12)/5(In5)
  tau_psi/1 -> S(10-12)/6(In6)
  S(10-12)/1(Out1) -> Mux/10
  S(10-12)/2(Out2) -> Mux/11
  S(10-12)/3(Out3) -> Mux/12
  Demux1/1 -> Terminator/1  "x"
  Demux1/2 -> Terminator1/1  "y"
  Demux1/3 -> Terminator2/1  "z"
  T/1 -> Gain/1  "z_ref"

== system Gen_net_5/quad 3/references ==
  From Workspace : FromWorkspace  VariableName=z_ref_3  SampleTime=0
  From Workspace1 : FromWorkspace  VariableName=x_ref_3  SampleTime=0
  From Workspace2 : FromWorkspace  VariableName=y_ref_3  SampleTime=0
  reference : Scope  NumInputPorts=3
  x_ref : Outport
  y_ref : Outport  Port=2
  z_ref : Outport  Port=3
  wires:
  From Workspace1/1 -> reference/1, x_ref/1  "x_ref"
  From Workspace/1 -> reference/3, z_ref/1  "z_ref"
  From Workspace2/1 -> reference/2, y_ref/1  "y_ref"

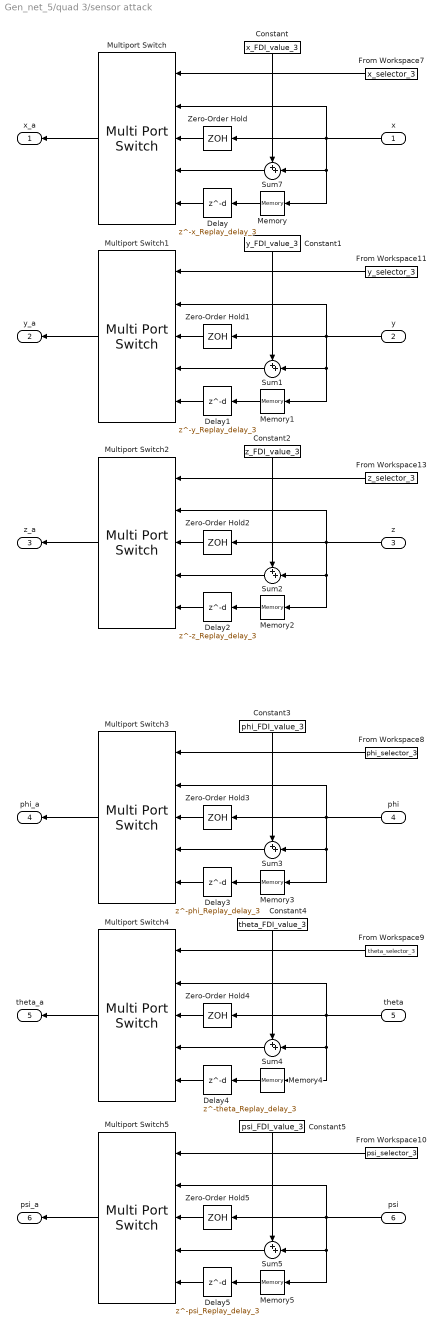
== system Gen_net_5/quad 3/sensor attack ==
  x : Inport
  y : Inport  Port=2
  z : Inport  Port=3
  phi : Inport  Port=4
  theta : Inport  Port=5
  psi : Inport  Port=6
  Constant : Constant  Value=x_FDI_value_3
  Constant1 : Constant  Value=y_FDI_value_3
  Constant2 : Constant  Value=z_FDI_value_3
  Constant3 : Constant  Value=phi_FDI_value_3
  Constant4 : Constant  Value=theta_FDI_value_3
  Constant5 : Constant  Value=psi_FDI_value_3
  Delay : Delay  DelayLength=x_Replay_delay_3  DelayLengthUpperLimit=40
  Delay1 : Delay  DelayLength=y_Replay_delay_3  DelayLengthUpperLimit=40
  Delay2 : Delay  DelayLength=z_Replay_delay_3  DelayLengthUpperLimit=40
  Delay3 : Delay  DelayLength=phi_Replay_delay_3  DelayLengthUpperLimit=40
  Delay4 : Delay  DelayLength=theta_Replay_delay_3  DelayLengthUpperLimit=40
  Delay5 : Delay  DelayLength=psi_Replay_delay_3  DelayLengthUpperLimit=40
  From Workspace10 : FromWorkspace  VariableName=psi_selector_3  SampleTime=0
  From Workspace11 : FromWorkspace  VariableName=y_selector_3  SampleTime=0
  From Workspace13 : FromWorkspace  VariableName=z_selector_3  SampleTime=0
  From Workspace7 : FromWorkspace  VariableName=x_selector_3  SampleTime=0
  From Workspace8 : FromWorkspace  VariableName=phi_selector_3  SampleTime=0
  From Workspace9 : FromWorkspace  VariableName=theta_selector_3  SampleTime=0
  Memory{,1..5} (6 alike) : Memory
  Multiport Switch{,1..5} (6 alike) : MultiPortSwitch  Inputs=4
  Sum{1..5,7} (6 alike) : Sum  Inputs=++|
  Zero-Order Hold : ZeroOrderHold  SampleTime=x_DoS_duration_3
  Zero-Order Hold1 : ZeroOrderHold  SampleTime=y_DoS_duration_3
  Zero-Order Hold2 : ZeroOrderHold  SampleTime=z_DoS_duration_3
  Zero-Order Hold3 : ZeroOrderHold  SampleTime=phi_DoS_duration_3
  Zero-Order Hold4 : ZeroOrderHold  SampleTime=theta_DoS_duration_3
  Zero-Order Hold5 : ZeroOrderHold  SampleTime=psi_DoS_duration_3
  x_a : Outport
  y_a : Outport  Port=2
  z_a : Outport  Port=3
  phi_a : Outport  Port=4
  theta_a : Outport  Port=5
  psi_a : Outport  Port=6
  wires:
  Memory/1 -> Delay/1
  Delay/1 -> Multiport Switch/5
  Zero-Order Hold/1 -> Multiport Switch/3
  Constant/1 -> Sum7/1
  Sum7/1 -> Multiport Switch/4
  Multiport Switch/1 -> x_a/1
  x/1 -> Multiport Switch/2, Zero-Order Hold/1, Sum7/2, Memory/1
  From Workspace7/1 -> Multiport Switch/1
  From Workspace11/1 -> Multiport Switch1/1
  Sum1/1 -> Multiport Switch1/4
  Delay1/1 -> Multiport Switch1/5
  Constant1/1 -> Sum1/1
  Memory1/1 -> Delay1/1
  y/1 -> Multiport Switch1/2, Zero-Order Hold1/1, Sum1/2, Memory1/1
  Multiport Switch1/1 -> y_a/1
  Zero-Order Hold1/1 -> Multiport Switch1/3
  From Workspace13/1 -> Multiport Switch2/1
  Sum2/1 -> Multiport Switch2/4
  Delay2/1 -> Multiport Switch2/5
  Constant2/1 -> Sum2/1
  Memory2/1 -> Delay2/1
  z/1 -> Multiport Switch2/2, Zero-Order Hold2/1, Sum2/2, Memory2/1
  Multiport Switch2/1 -> z_a/1
  Zero-Order Hold2/1 -> Multiport Switch2/3
  From Workspace8/1 -> Multiport Switch3/1
  Sum3/1 -> Multiport Switch3/4
  Delay3/1 -> Multiport Switch3/5
  Constant3/1 -> Sum3/1
  Memory3/1 -> Delay3/1
  phi/1 -> Multiport Switch3/2, Zero-Order Hold3/1, Sum3/2, Memory3/1
  Multiport Switch3/1 -> phi_a/1
  Zero-Order Hold3/1 -> Multiport Switch3/3
  From Workspace9/1 -> Multiport Switch4/1
  Sum4/1 -> Multiport Switch4/4
  Delay4/1 -> Multiport Switch4/5
  Constant4/1 -> Sum4/1
  Memory4/1 -> Delay4/1
  theta/1 -> Multiport Switch4/2, Zero-Order Hold4/1, Sum4/2, Memory4/1
  Multiport Switch4/1 -> theta_a/1
  Zero-Order Hold4/1 -> Multiport Switch4/3
  From Workspace10/1 -> Multiport Switch5/1
  Sum5/1 -> Multiport Switch5/4
  Delay5/1 -> Multiport Switch5/5
  Constant5/1 -> Sum5/1
  Memory5/1 -> Delay5/1
  psi/1 -> Multiport Switch5/2, Zero-Order Hold5/1, Sum5/2, Memory5/1
  Multiport Switch5/1 -> psi_a/1
  Zero-Order Hold5/1 -> Multiport Switch5/3

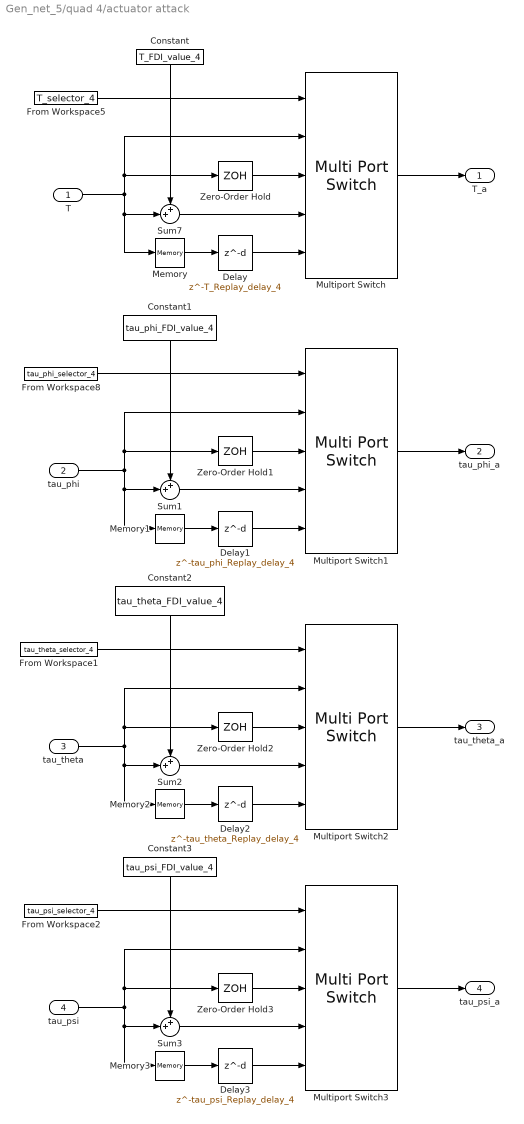
== system Gen_net_5/quad 4/actuator attack ==
  T : Inport
  tau_phi : Inport  Port=2
  tau_theta : Inport  Port=3
  tau_psi : Inport  Port=4
  Constant : Constant  Value=T_FDI_value_4
  Constant1 : Constant  Value=tau_phi_FDI_value_4
  Constant2 : Constant  Value=tau_theta_FDI_value_4
  Constant3 : Constant  Value=tau_psi_FDI_value_4
  Delay : Delay  DelayLength=T_Replay_delay_4  DelayLengthUpperLimit=40
  Delay1 : Delay  DelayLength=tau_phi_Replay_delay_4  DelayLengthUpperLimit=40
  Delay2 : Delay  DelayLength=tau_theta_Replay_delay_4  DelayLengthUpperLimit=40
  Delay3 : Delay  DelayLength=tau_psi_Replay_delay_4  DelayLengthUpperLimit=40
  From Workspace1 : FromWorkspace  VariableName=tau_theta_selector_4  SampleTime=0
  From Workspace2 : FromWorkspace  VariableName=tau_psi_selector_4  SampleTime=0
  From Workspace5 : FromWorkspace  VariableName=T_selector_4  SampleTime=0
  From Workspace8 : FromWorkspace  VariableName=tau_phi_selector_4  SampleTime=0
  Memory{,1..3} (4 alike) : Memory
  Multiport Switch{,1..3} (4 alike) : MultiPortSwitch  Inputs=4
  Sum{1..3,7} (4 alike) : Sum  Inputs=++|
  Zero-Order Hold : ZeroOrderHold  SampleTime=T_DoS_duration_4
  Zero-Order Hold1 : ZeroOrderHold  SampleTime=tau_phi_DoS_duration_4
  Zero-Order Hold2 : ZeroOrderHold  SampleTime=tau_theta_DoS_duration_4
  Zero-Order Hold3 : ZeroOrderHold  SampleTime=tau_psi_DoS_duration_4
  T_a : Outport
  tau_phi_a : Outport  Port=2
  tau_theta_a : Outport  Port=3
  tau_psi_a : Outport  Port=4
  wires:
  T/1 -> Sum7/2, Memory/1, Multiport Switch/2, Zero-Order Hold/1
  Zero-Order Hold/1 -> Multiport Switch/3
  Sum7/1 -> Multiport Switch/4
  From Workspace5/1 -> Multiport Switch/1
  Multiport Switch/1 -> T_a/1
  Memory/1 -> Delay/1
  Constant/1 -> Sum7/1
  Delay/1 -> Multiport Switch/5
  Memory1/1 -> Delay1/1
  Delay1/1 -> Multiport Switch1/5
  Zero-Order Hold1/1 -> Multiport Switch1/3
  Constant1/1 -> Sum1/1
  Sum1/1 -> Multiport Switch1/4
  Multiport Switch1/1 -> tau_phi_a/1
  tau_phi/1 -> Sum1/2, Memory1/1, Multiport Switch1/2, Zero-Order Hold1/1
  From Workspace8/1 -> Multiport Switch1/1
  Memory2/1 -> Delay2/1
  Delay2/1 -> Multiport Switch2/5
  Zero-Order Hold2/1 -> Multiport Switch2/3
  Constant2/1 -> Sum2/1
  Sum2/1 -> Multiport Switch2/4
  Multiport Switch2/1 -> tau_theta_a/1
  tau_theta/1 -> Sum2/2, Memory2/1, Multiport Switch2/2, Zero-Order Hold2/1
  From Workspace1/1 -> Multiport Switch2/1
  Memory3/1 -> Delay3/1
  Delay3/1 -> Multiport Switch3/5
  Zero-Order Hold3/1 -> Multiport Switch3/3
  Constant3/1 -> Sum3/1
  Sum3/1 -> Multiport Switch3/4
  Multiport Switch3/1 -> tau_psi_a/1
  tau_psi/1 -> Sum3/2, Memory3/1, Multiport Switch3/2, Zero-Order Hold3/1
  From Workspace2/1 -> Multiport Switch3/1

== system Gen_net_5/quad 4/controller ==
  x_ref : Inport
  y_ref : Inport  Port=2
  z_ref : Inport  Port=3
  x : Inport  Port=4
  y : Inport  Port=5
  z : Inport  Port=6
  phi : Inport  Port=7
  theta : Inport  Port=8
  psi : Inport  Port=9
  altitude controller : Subsystem
  attitude controller : Subsystem
  position controller : Subsystem
  yaw controller : Subsystem
  T : Outport
  tau_phi : Outport  Port=2
  tau_theta : Outport  Port=3
  tau_psi : Outport  Port=4
  wires:
  yaw controller/1(tau_psi) -> tau_psi/1
  phi/1 -> attitude controller/1(phi)
  y_ref/1 -> position controller/3(y_ref)
  x/1 -> position controller/2(x)
  position controller/2(theta_ref) -> attitude controller/4(theta_ref)
  position controller/1(phi_ref) -> attitude controller/3(phi_ref)
  x_ref/1 -> position controller/1(x_ref)
  attitude controller/1(tau_phi) -> tau_phi/1
  y/1 -> position controller/4(y)
  psi/1 -> yaw controller/1(yaw)
  attitude controller/2(tau_theta) -> tau_theta/1
  theta/1 -> attitude controller/2(theta)
  z_ref/1 -> altitude controller/1(z_ref)
  altitude controller/1(T) -> T/1
  z/1 -> altitude controller/2(z)

== system Gen_net_5/quad 4/quadcopter ==
  T : Inport
  tau_ phi : Inport  Port=2
  tau_theta : Inport  Port=3
  tau_psi : Inport  Port=4
  Demux : Demux  Outputs=12
  Demux1 : Demux  Outputs=12
  Gain : Gain  Gain=1/m
  Integrator12 : Integrator
  Mux : Mux  Inputs=12
  S(10-12) : Subsystem
  S(4-6) : Subsystem
  S(7-9) : Subsystem
  Scope1 : Scope  NumInputPorts=3
  Scope2 : Scope  NumInputPorts=3
  Terminator : Terminator
  Terminator1 : Terminator
  Terminator2 : Terminator
  angle : Scope  NumInputPorts=3
  position : Scope  NumInputPorts=3
  x : Outport
  y : Outport  Port=2
  z : Outport  Port=3
  phi : Outport  Port=4
  theta : Outport  Port=5
  psi : Outport  Port=6
  wires:
  Mux/1 -> Integrator12/1
  Integrator12/1 -> Demux/1, Demux1/1
  Demux/2 -> position/2, y/1  "y"
  Demux/3 -> z/1, position/3  "z"
  Demux/1 -> x/1, position/1  "x"
  Demux/5 -> Scope1/2  "Vy"
  Demux/4 -> Scope1/1  "Vx"
  Demux/6 -> Scope1/3  "Vz"
  Demux/8 -> angle/2, theta/1  "theta"
  Demux/7 -> angle/1, phi/1  "phi"
  Demux/9 -> angle/3, psi/1  "psi"
  Demux/12 -> Scope2/3  "r"
  Demux/10 -> Scope2/1  "p"
  Demux/11 -> Scope2/2  "q"
  Demux1/4 -> Mux/1  "Vx"
  Demux1/5 -> Mux/2  "Vy"
  Demux1/6 -> Mux/3  "Vz"
  Demux1/8 -> S(4-6)/3(theta), S(7-9)/2(theta)  "theta"
  Demux1/7 -> S(4-6)/2(phi), S(7-9)/1(phi)  "phi"
  Demux1/10 -> S(10-12)/2(P), S(7-9)/4(P)  "P"
  Demux1/11 -> S(7-9)/3(q), S(10-12)/1(q)  "q"
  Demux1/12 -> S(7-9)/5(r), S(10-12)/3(r)
  Gain/1 -> S(4-6)/1(In1)
  Demux1/9 -> S(4-6)/4(psi)  "psi"
  S(4-6)/1(Out1) -> Mux/4
  S(4-6)/2(Out2) -> Mux/5
  S(4-6)/3(Out3) -> Mux/6
  S(7-9)/1(Out1) -> Mux/7
  S(7-9)/2(Out2) -> Mux/8
  S(7-9)/3(Out3) -> Mux/9
  tau_ phi/1 -> S(10-12)/4(In4)
  tau_theta/1 -> S(10-12)/5(In5)
  tau_psi/1 -> S(10-12)/6(In6)
  S(10-12)/1(Out1) -> Mux/10
  S(10-12)/2(Out2) -> Mux/11
  S(10-12)/3(Out3) -> Mux/12
  Demux1/1 -> Terminator/1  "x"
  Demux1/2 -> Terminator1/1  "y"
  Demux1/3 -> Terminator2/1  "z"
  T/1 -> Gain/1  "z_ref"

== system Gen_net_5/quad 4/references ==
  From Workspace : FromWorkspace  VariableName=z_ref_4  SampleTime=0
  From Workspace1 : FromWorkspace  VariableName=x_ref_4  SampleTime=0
  From Workspace2 : FromWorkspace  VariableName=y_ref_4  SampleTime=0
  reference : Scope  NumInputPorts=3
  x_ref : Outport
  y_ref : Outport  Port=2
  z_ref : Outport  Port=3
  wires:
  From Workspace1/1 -> reference/1, x_ref/1  "x_ref"
  From Workspace/1 -> reference/3, z_ref/1  "z_ref"
  From Workspace2/1 -> reference/2, y_ref/1  "y_ref"

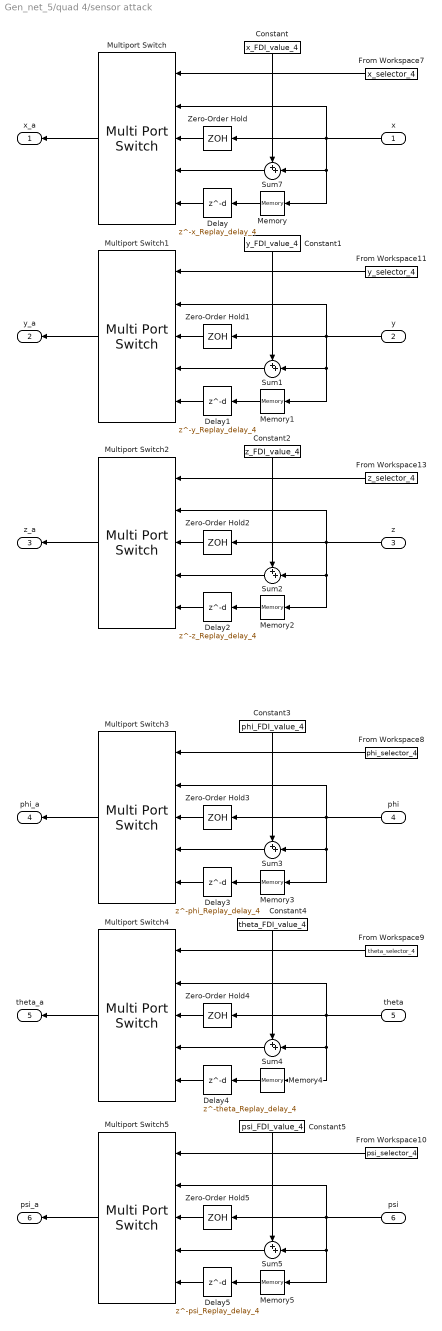
== system Gen_net_5/quad 4/sensor attack ==
  x : Inport
  y : Inport  Port=2
  z : Inport  Port=3
  phi : Inport  Port=4
  theta : Inport  Port=5
  psi : Inport  Port=6
  Constant : Constant  Value=x_FDI_value_4
  Constant1 : Constant  Value=y_FDI_value_4
  Constant2 : Constant  Value=z_FDI_value_4
  Constant3 : Constant  Value=phi_FDI_value_4
  Constant4 : Constant  Value=theta_FDI_value_4
  Constant5 : Constant  Value=psi_FDI_value_4
  Delay : Delay  DelayLength=x_Replay_delay_4  DelayLengthUpperLimit=40
  Delay1 : Delay  DelayLength=y_Replay_delay_4  DelayLengthUpperLimit=40
  Delay2 : Delay  DelayLength=z_Replay_delay_4  DelayLengthUpperLimit=40
  Delay3 : Delay  DelayLength=phi_Replay_delay_4  DelayLengthUpperLimit=40
  Delay4 : Delay  DelayLength=theta_Replay_delay_4  DelayLengthUpperLimit=40
  Delay5 : Delay  DelayLength=psi_Replay_delay_4  DelayLengthUpperLimit=40
  From Workspace10 : FromWorkspace  VariableName=psi_selector_4  SampleTime=0
  From Workspace11 : FromWorkspace  VariableName=y_selector_4  SampleTime=0
  From Workspace13 : FromWorkspace  VariableName=z_selector_4  SampleTime=0
  From Workspace7 : FromWorkspace  VariableName=x_selector_4  SampleTime=0
  From Workspace8 : FromWorkspace  VariableName=phi_selector_4  SampleTime=0
  From Workspace9 : FromWorkspace  VariableName=theta_selector_4  SampleTime=0
  Memory{,1..5} (6 alike) : Memory
  Multiport Switch{,1..5} (6 alike) : MultiPortSwitch  Inputs=4
  Sum{1..5,7} (6 alike) : Sum  Inputs=++|
  Zero-Order Hold : ZeroOrderHold  SampleTime=x_DoS_duration_4
  Zero-Order Hold1 : ZeroOrderHold  SampleTime=y_DoS_duration_4
  Zero-Order Hold2 : ZeroOrderHold  SampleTime=z_DoS_duration_4
  Zero-Order Hold3 : ZeroOrderHold  SampleTime=phi_DoS_duration_4
  Zero-Order Hold4 : ZeroOrderHold  SampleTime=theta_DoS_duration_4
  Zero-Order Hold5 : ZeroOrderHold  SampleTime=psi_DoS_duration_4
  x_a : Outport
  y_a : Outport  Port=2
  z_a : Outport  Port=3
  phi_a : Outport  Port=4
  theta_a : Outport  Port=5
  psi_a : Outport  Port=6
  wires:
  Memory/1 -> Delay/1
  Delay/1 -> Multiport Switch/5
  Zero-Order Hold/1 -> Multiport Switch/3
  Constant/1 -> Sum7/1
  Sum7/1 -> Multiport Switch/4
  Multiport Switch/1 -> x_a/1
  x/1 -> Multiport Switch/2, Zero-Order Hold/1, Sum7/2, Memory/1
  From Workspace7/1 -> Multiport Switch/1
  From Workspace11/1 -> Multiport Switch1/1
  Sum1/1 -> Multiport Switch1/4
  Delay1/1 -> Multiport Switch1/5
  Constant1/1 -> Sum1/1
  Memory1/1 -> Delay1/1
  y/1 -> Multiport Switch1/2, Zero-Order Hold1/1, Sum1/2, Memory1/1
  Multiport Switch1/1 -> y_a/1
  Zero-Order Hold1/1 -> Multiport Switch1/3
  From Workspace13/1 -> Multiport Switch2/1
  Sum2/1 -> Multiport Switch2/4
  Delay2/1 -> Multiport Switch2/5
  Constant2/1 -> Sum2/1
  Memory2/1 -> Delay2/1
  z/1 -> Multiport Switch2/2, Zero-Order Hold2/1, Sum2/2, Memory2/1
  Multiport Switch2/1 -> z_a/1
  Zero-Order Hold2/1 -> Multiport Switch2/3
  From Workspace8/1 -> Multiport Switch3/1
  Sum3/1 -> Multiport Switch3/4
  Delay3/1 -> Multiport Switch3/5
  Constant3/1 -> Sum3/1
  Memory3/1 -> Delay3/1
  phi/1 -> Multiport Switch3/2, Zero-Order Hold3/1, Sum3/2, Memory3/1
  Multiport Switch3/1 -> phi_a/1
  Zero-Order Hold3/1 -> Multiport Switch3/3
  From Workspace9/1 -> Multiport Switch4/1
  Sum4/1 -> Multiport Switch4/4
  Delay4/1 -> Multiport Switch4/5
  Constant4/1 -> Sum4/1
  Memory4/1 -> Delay4/1
  theta/1 -> Multiport Switch4/2, Zero-Order Hold4/1, Sum4/2, Memory4/1
  Multiport Switch4/1 -> theta_a/1
  Zero-Order Hold4/1 -> Multiport Switch4/3
  From Workspace10/1 -> Multiport Switch5/1
  Sum5/1 -> Multiport Switch5/4
  Delay5/1 -> Multiport Switch5/5
  Constant5/1 -> Sum5/1
  Memory5/1 -> Delay5/1
  psi/1 -> Multiport Switch5/2, Zero-Order Hold5/1, Sum5/2, Memory5/1
  Multiport Switch5/1 -> psi_a/1
  Zero-Order Hold5/1 -> Multiport Switch5/3
